simulink model "lec11_slides_ex2"  (R2023b)
settings: Solver=VariableStepAuto  StartTime=0.0  StopTime=2  RelTol=1e-3
libraries: simulink_extras x2
settings Model: Creator=john  LastModifiedBy=john

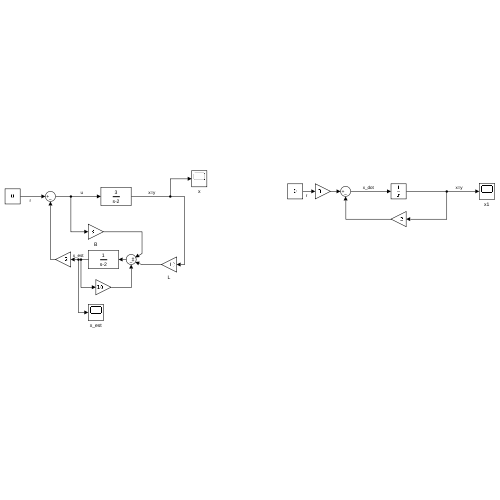
[thumbnail: Simulink's stored preview of the top-level diagram]
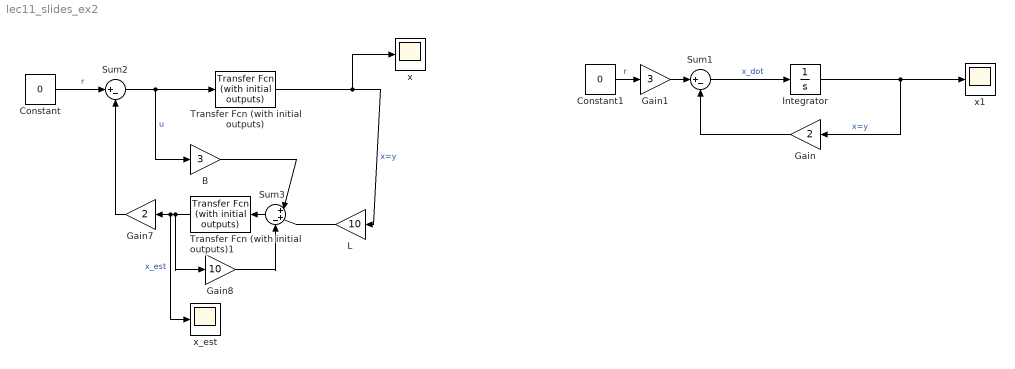
== system lec11_slides_ex2 ==
  B : Gain  Gain=3
  Constant : Constant  Value=0
  Constant1 : Constant  Value=0
  Gain : Gain  Gain=2
  Gain1 : Gain  Gain=3
  Gain7 : Gain  Gain=2
  Gain8 : Gain  Gain=10
  Integrator : Integrator  InitialCondition=1
  L : Gain  Gain=10
  Sum1 : Sum  Inputs=|+-
  Sum2 : Sum  Inputs=|+-
  Sum3 : Sum  Inputs=|++-
  Transfer Fcn (with initial outputs) : simulink_extras/Additional Linear/Transfer Fcn (with initial outputs)  N=[3]  D=[1 -2]  Y0=1  U0=0
  Transfer Fcn (with initial outputs)1 : simulink_extras/Additional Linear/Transfer Fcn (with initial outputs)  N=[1]  D=[1 -2]  Y0=0  U0=0
  x : Scope
  x1 : Scope
  x_est : Scope
  wires:
  Constant/1 -> Sum2/1  "r"
  Gain7/1 -> Sum2/2
  Sum2/1 -> Transfer Fcn (with initial outputs)/1, B/1  "u"
  Transfer Fcn (with initial outputs)/1 -> x/1, L/1  "x=y"
  L/1 -> Sum3/2
  B/1 -> Sum3/1
  Sum3/1 -> Transfer Fcn (with initial outputs)1/1
  Transfer Fcn (with initial outputs)1/1 -> Gain8/1, x_est/1, Gain7/1  "x_est"
  Gain8/1 -> Sum3/3
  Constant1/1 -> Gain1/1  "r"
  Sum1/1 -> Integrator/1  "x_dot"
  Integrator/1 -> Gain/1, x1/1  "x=y"
  Gain/1 -> Sum1/2
  Gain1/1 -> Sum1/1
